simulink model "elevator"  (R2019b)
settings: Solver=FixedStepAuto  StartTime=0.0  StopTime=10.0  RelTol=1e-3
libraries: eePwmGenerator x2
settings Model: ExtModeTrigDuration=2  Creator=sin29  LastModifiedBy=mr
settings DataIOCC: ReturnWorkspaceOutputs=off
settings OptimizationCC: DefaultParameterBehavior=Inlined  UseDivisionForNetSlopeComputation=on  UseFloatMulNetSlope=on  InlineInvariantSignals=on  PassReuseOutputArgsAs=Individual arguments  ZeroExternalMemoryAtStartup=off  ZeroInternalMemoryAtStartup=off  NoFixptDivByZeroProtection=on  EfficientFloat2IntCast=on  LifeSpan=1  MaxStackSize=64  OptimizeBlockOrder=speed  DifferentSizesBufferReuse=on  EfficientTunableParamExpr=on
settings DebuggingCC: ParameterTunabilityLossMsg=error  ArithmeticOperatorsInVariantConditions=warning
settings HardwareCC: ProdBitPerInt=16  ProdBitPerPointer=16  ProdBitPerSizeT=16  ProdBitPerPtrDiffT=16  ProdLargestAtomicFloat=None  ProdWordSize=8  ProdLongLongMode=on  ProdHWDeviceType=Atmel->AVR
settings SFSimCC: MATLABDynamicMemAlloc=off  CustomCodeUndefinedFunction=UseInterfaceOnly
settings RTWCC: SystemTargetFile=ert.tlc  HardwareBoard=Arduino Uno  TLCOptions=-aInlineSetEventsForThisBaseRateFcn=TLC_FALSE -aSuppressMultiTaskScheduler=TLC_FALSE -aRateBasedStepFcn=1  GenCodeOnly=on  TemplateMakefile=ert_default_tmf  GenerateReport=on  Toolchain=Arduino AVR  BuildConfiguration=Faster Runs  IncludeHyperlinkInReport=on  LaunchReport=on  GenerateTraceInfo=on  GenerateTraceReport=on  GenerateTraceReportSl=on  GenerateTraceReportSf=on  GenerateTraceReportEml=on  GenerateCodeMetricsReport=on
settings CodeAppCC: ForceParamTrailComments=on  IgnoreCustomStorageClasses=off  OperatorAnnotations=on  SimulinkDataObjDesc=on  SFDataObjDesc=on  CustomSymbolStrGlobalVar=rt$N$M  CustomSymbolStrType=$N$M  CustomSymbolStrFcn=$N$M$F  CustomSymbolStrMacro=$N$M  InsertBlockDesc=on
settings ERTTargetCC: IncludeMdlTerminateFcn=off  CombineSignalStateStructs=on  SupportAbsoluteTime=off  SupportComplex=off  SupportNonInlinedSFcns=on  InlinedParameterPlacement=NonHierarchical  ERTFilePackagingFormat=CompactWithDataFile

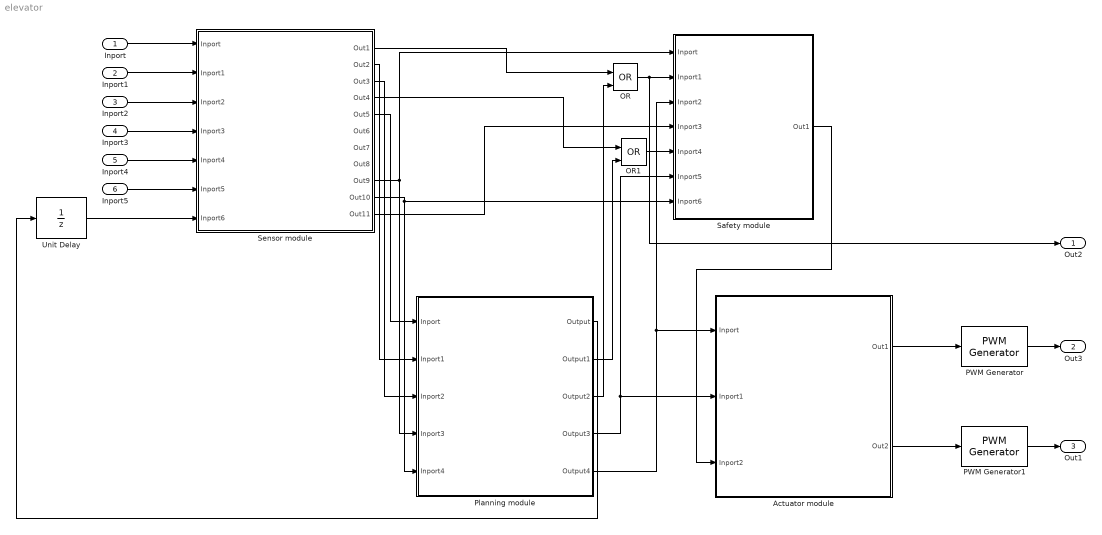
== system elevator ==
  Inport : Inport
  Inport1 : Inport  Port=2
  Inport2 : Inport  Port=3
  Inport3 : Inport  Port=4
  Inport4 : Inport  Port=5
  Inport5 : Inport  Port=6
  Actuator module : Subsystem
  OR : Logic  Operator=OR  IconShape=distinctive  AllPortsSameDT=off  OutDataTypeStr=boolean
  OR1 : Logic  Operator=OR  IconShape=distinctive  AllPortsSameDT=off  OutDataTypeStr=boolean
  PWM Generator : eePwmGenerator/PWM Generator  CarrCount=Up  Tper=0.001  Ts=5e-5
      settings: SourceProductName=Simscape Electrical
  PWM Generator1 : eePwmGenerator/PWM Generator  CarrCount=Up  Tper=0.001  Ts=5e-5
      settings: SourceProductName=Simscape Electrical
  Planning module : Subsystem
  Safety module : Subsystem
  Sensor module : Subsystem
  Unit Delay : UnitDelay  SampleTime=-1  HasFrameUpgradeWarning=on
  Out2 : Outport
  Out3 : Outport  Port=2
  Out1 : Outport  Port=3
  wires:
  Inport3/1 -> Sensor module/4(Inport3)
  Inport4/1 -> Sensor module/5(Inport4)
  Inport5/1 -> Sensor module/6(Inport5)
  Inport1/1 -> Sensor module/2(Inport1)
  Inport/1 -> Sensor module/1(Inport)
  Inport2/1 -> Sensor module/3(Inport2)
  Sensor module/4(Out4) -> OR1/1
  Sensor module/5(Out5) -> Planning module/1(Inport)
  Sensor module/2(Out2) -> Planning module/2(Inport1)
  Sensor module/3(Out3) -> Planning module/3(Inport2)
  Sensor module/10(Out10) -> Safety module/7(Inport6), Planning module/5(Inport4)
  Sensor module/9(Out9) -> Safety module/1(Inport), Planning module/4(Inport3)
  Unit Delay/1 -> Sensor module/7(Inport6)
  Planning module/1(Output) -> Unit Delay/1
  Sensor module/11(Out11) -> Safety module/4(Inport3)
  Sensor module/1(Out1) -> OR/1
  OR/1 -> Safety module/2(Inport1), Out2/1
  Planning module/3(Output2) -> OR/2
  OR1/1 -> Safety module/5(Inport4)
  Planning module/2(Output1) -> OR1/2
  Planning module/4(Output3) -> Actuator module/2(Inport1), Safety module/6(Inport5)
  Planning module/5(Output4) -> Actuator module/1(Inport), Safety module/3(Inport2)
  PWM Generator/1 -> Out3/1
  PWM Generator1/1 -> Out1/1
  Safety module/1(Out1) -> Actuator module/3(Inport2)
  Actuator module/1(Out1) -> PWM Generator/1
  Actuator module/2(Out2) -> PWM Generator1/1

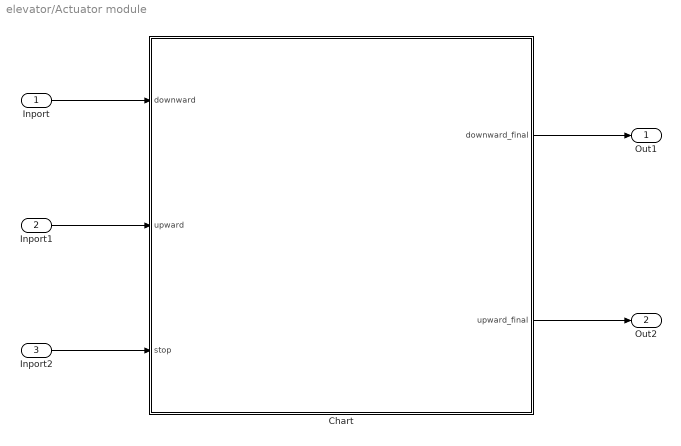
== system elevator/Actuator module ==
  Inport : Inport
  Inport1 : Inport  Port=2
  Inport2 : Inport  Port=3
  Chart : Stateflow chart  BlockKeywords=__PRM__SERIALIZED__DATA__:Stateflow Chart,Stateflow Diagram  TreatAsAtomicUnit=on
  Out1 : Outport
  Out2 : Outport  Port=2
  wires:
  Inport/1 -> Chart/1(downward)
  Inport1/1 -> Chart/2(upward)
  Inport2/1 -> Chart/3(stop)
  Chart/1(downward_final) -> Out1/1
  Chart/2(upward_final) -> Out2/1

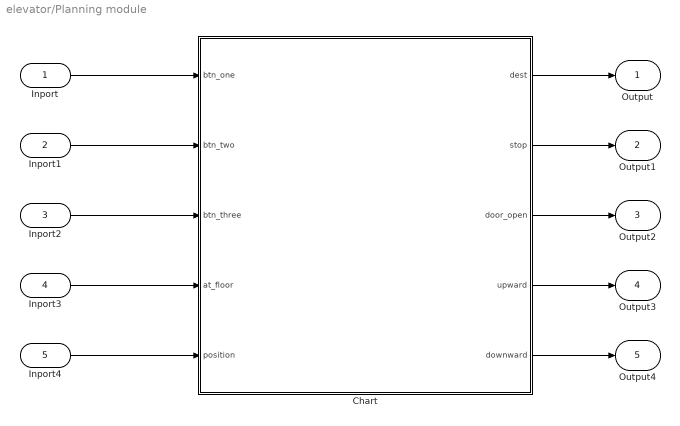
== system elevator/Planning module ==
  Inport : Inport
  Inport1 : Inport  Port=2
  Inport2 : Inport  Port=3
  Inport3 : Inport  Port=4
  Inport4 : Inport  Port=5
  Chart : Stateflow chart  BlockKeywords=__PRM__SERIALIZED__DATA__:Stateflow Chart,Stateflow Diagram  TreatAsAtomicUnit=on
  Output : Outport
  Output1 : Outport  Port=2
  Output2 : Outport  Port=3
  Output3 : Outport  Port=4
  Output4 : Outport  Port=5
  wires:
  Inport/1 -> Chart/1(btn_one)
  Inport4/1 -> Chart/5(position)
  Inport3/1 -> Chart/4(at_floor)
  Inport2/1 -> Chart/3(btn_three)
  Inport1/1 -> Chart/2(btn_two)
  Chart/1(dest) -> Output/1
  Chart/2(stop) -> Output1/1
  Chart/3(door_open) -> Output2/1
  Chart/5(downward) -> Output4/1
  Chart/4(upward) -> Output3/1

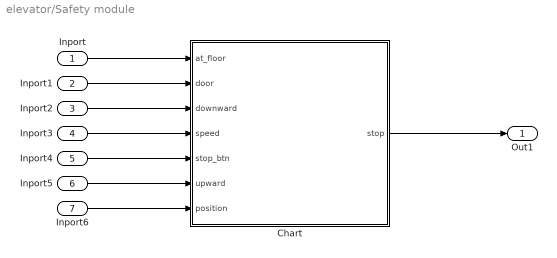
== system elevator/Safety module ==
  Inport : Inport
  Inport1 : Inport  Port=2
  Inport2 : Inport  Port=3
  Inport3 : Inport  Port=4
  Inport4 : Inport  Port=5
  Inport5 : Inport  Port=6
  Inport6 : Inport  Port=7
  Chart : Stateflow chart  TreatAsAtomicUnit=on
  Out1 : Outport  VectorParamsAs1DForOutWhenUnconnected=off
  wires:
  Inport/1 -> Chart/1(at_floor)
  Inport1/1 -> Chart/2(door)
  Inport2/1 -> Chart/3(downward)
  Inport3/1 -> Chart/4(speed)
  Inport4/1 -> Chart/5(stop_btn)
  Inport5/1 -> Chart/6(upward)
  Chart/1(stop) -> Out1/1
  Inport6/1 -> Chart/7(position)

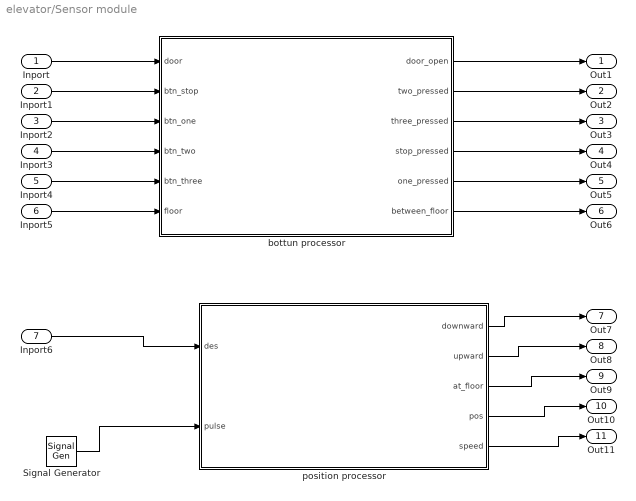
== system elevator/Sensor module ==
  Inport : Inport
  Inport1 : Inport  Port=2
  Inport2 : Inport  Port=3
  Inport3 : Inport  Port=4
  Inport4 : Inport  Port=5
  Inport5 : Inport  Port=6
  Inport6 : Inport  Port=7
  Signal Generator : SignalGenerator  Units=rad/sec
  "bottun processor " : Stateflow chart  TreatAsAtomicUnit=on
  "position processor " : Stateflow chart  TreatAsAtomicUnit=on
  Out1 : Outport  VectorParamsAs1DForOutWhenUnconnected=off
  Out2 : Outport  Port=2  VectorParamsAs1DForOutWhenUnconnected=off
  Out3 : Outport  Port=3  VectorParamsAs1DForOutWhenUnconnected=off
  Out4 : Outport  Port=4  VectorParamsAs1DForOutWhenUnconnected=off
  Out5 : Outport  Port=5  VectorParamsAs1DForOutWhenUnconnected=off
  Out6 : Outport  Port=6  VectorParamsAs1DForOutWhenUnconnected=off
  Out7 : Outport  Port=7  VectorParamsAs1DForOutWhenUnconnected=off
  Out8 : Outport  Port=8  VectorParamsAs1DForOutWhenUnconnected=off
  Out9 : Outport  Port=9  VectorParamsAs1DForOutWhenUnconnected=off
  Out10 : Outport  Port=10  VectorParamsAs1DForOutWhenUnconnected=off
  Out11 : Outport  Port=11  VectorParamsAs1DForOutWhenUnconnected=off
  wires:
  Inport/1 -> "bottun processor "/1(door)
  Inport1/1 -> "bottun processor "/2(btn_stop)
  Inport2/1 -> "bottun processor "/3(btn_one)
  Inport3/1 -> "bottun processor "/4(btn_two)
  Inport4/1 -> "bottun processor "/5(btn_three)
  Inport5/1 -> "bottun processor "/6(floor)
  Inport6/1 -> "position processor "/1(des)
  Signal Generator/1 -> "position processor "/2(pulse)
  "bottun processor "/1(door_open) -> Out1/1
  "bottun processor "/2(two_pressed) -> Out2/1
  "bottun processor "/3(three_pressed) -> Out3/1
  "bottun processor "/4(stop_pressed) -> Out4/1
  "bottun processor "/5(one_pressed) -> Out5/1
  "bottun processor "/6(between_floor) -> Out6/1
  "position processor "/1(downward) -> Out7/1
  "position processor "/2(upward) -> Out8/1
  "position processor "/3(at_floor) -> Out9/1
  "position processor "/4(pos) -> Out10/1
  "position processor "/5(speed) -> Out11/1

== stateflow chart elevator/Sensor module/position processor  ==
  state pos_detection
    state speed_cal [parallel]
      settings: executionOrder=1
      state speed_at_1
        entry:
        speed = (pos  - last_counter);
        last_counter = pos;
      (default) -> speed_at_1
      speed_at_1 -> speed_at_1 : [after(1,sec)]
    state pos_cal [parallel]
      settings: executionOrder=2
      (history)
      state floor_1
        entry:
        counter = 0;
        at_floor = 1;
        pos = 0;
        during:
        upward = 0;
        downward = 0;
      state floor_3
        entry:
        counter = 0;
        at_floor = 3;
        pos = 800;
        during:
        upward = 0;
        downward = 0;
      state between_1_2
        entry:
        at_floor = -1;
        pos = (upward)*(counter) + (downward)*(400 - counter)
        exit:
      state between_2_3
        entry:
        at_floor = -1;
        pos = (upward)*(counter+400) + (downward)*(800 - counter)
      state read_pulse_2_3
        entry:
        counter = counter+1
        last = pulse;
      state read_pulse_1_2
        entry:
        counter = counter+1
        last = pulse
      state floor_2
        entry:
        counter = 0;
        at_floor = 2;
        pos  = 400;
        during:
        upward = 0;
        downward = 0;
      read_pulse_1_2 -> floor_1 [order 1] : [counter == 400 && downward == 1]
      read_pulse_2_3 -> floor_3 [order 1] : [counter == 400 && upward == 1]
      floor_1 -> between_1_2 : [des == 2 || des == 3]{upward = 1;downward = 0}
      floor_3 -> between_2_3 : [des == 2 || des == 1]{upward = 0 ; downward = 1}
      between_1_2 -> between_1_2 [order 2] : [after(3,msec)&&last == pulse]
      read_pulse_1_2 -> between_1_2 [order 3] : [counter ~= 400]
      floor_2 -> between_2_3 [order 2] : [des == 3]{upward = 1; downward = 0}
      read_pulse_2_3 -> between_2_3 [order 3] : [counter ~= 400]
      between_2_3 -> read_pulse_2_3 : [after(3,msec)&& last ~= pulse]
      between_1_2 -> read_pulse_1_2 [order 1] : [after(3,msec)&& last ~= pulse]
      floor_2 -> between_1_2 [order 1] : [des == 1]{upward = 0;downward =1;}
      read_pulse_2_3 -> floor_2 [order 2] : [counter == 400 && downward == 1]
      read_pulse_1_2 -> floor_2 [order 2] : [counter == 400 && upward == 1]
    (default) -> floor_1
  state init
    exit :
    counter = 0;
    last_counter = 0;
    pos = 0;
  (default) -> init
  init -> pos_detection
  data: des input; pulse input; counter local; downward output; upward output; last local; at_floor output; pos output; speed output; last_counter local

== stateflow chart elevator/Safety module/Chart ==
  state down_stop
    entry :
    stop = 1;
  state both_dir_stop
    entry:
    stop = 1;
  state monitor
    during:
    stop = 0;
  state door_stop
    entry :
    stop = 1;
  state stop_button
    entry :
    stop = 1;
  state speed_stop
    entry :
    stop = 1;
  state top_stop
    entry :
    stop = 1;
  down_stop -> down_stop [order 1] : [after (10, msec) && position == 800 && at_floor == -1 && upward == 1]
  down_stop -> monitor [order 2] : [after (10, msec)  &&( at_floor ~= -1 || downward == 0)]
  monitor -> down_stop [order 5] : [after (10, msec) && position == 0 && at_floor == -1 && downward == 1]
  (default) -> monitor
  both_dir_stop -> both_dir_stop [order 2] : [after(10, msec) && upward == 1 && downward == 1]
  both_dir_stop -> monitor [order 1] : [after(10, msec) && (upward == 0 || downward == 0)]
  monitor -> both_dir_stop [order 6] : [after(10, msec) && upward == 1 && downward == 1]
  monitor -> top_stop [order 3] : [after (10, msec) && position == 800 && at_floor == -1 && upward == 1]
  monitor -> door_stop [order 1] : [after(10, msec) && door == 1 && at_floor ==-1]
  door_stop -> monitor [order 2] : [after(3, msec) && door == 0]
  top_stop -> monitor [order 1] : [after (10, msec)  &&( at_floor ~= -1 || upward == 0)]
  monitor -> stop_button [order 2] : [after (10, msec) && stop_btn == 1]
  stop_button -> monitor [order 2] : [after(3, msec) && stop_btn == 0]
  speed_stop -> monitor [order 1] : [after (10, msec) && speed <= 50]
  monitor -> speed_stop [order 4] : [after (10, msec) && speed > 50]
  door_stop -> door_stop [order 1] : [after(3, msec) && door == 1]
  stop_button -> stop_button [order 1] : [after(3, msec) && stop_btn == 1]
  speed_stop -> speed_stop [order 2] : [after (10, msec) && speed > 50]
  top_stop -> top_stop [order 2] : [after (10, msec) && position == 800 && at_floor == -1 && upward == 1]
  data: at_floor input; door input; downward input; speed input; stop_btn input; upward input; stop output; position input

== stateflow chart elevator/Sensor module/bottun processor  ==
  state Reset
    entry:
    one_pressed = 0;
    two_pressed = 0;
    three_pressed = 0;
    door_open = 0;
    stop_pressed = 0;
  state two_bounce
  state three_bounce
  state stop_bounce
  state one_bounce
  state door_bounce
  state floor_bounce
  state floor_pos
    entry :
    between_floor = 1;
  state two_press
    entry:
    two_pressed = 1;
  state stop_press
    entry:
    stop_pressed =1 ;
  state three_press
    entry:
    three_pressed = 1;
  state door_status
    entry:
    door_open = 1;
  state one_press
    entry:
    one_pressed = 1;
  floor_pos -> Reset
  floor_bounce -> Reset [order 1] : [floor == 0]
  Reset -> floor_bounce [order 6] : [floor == 1]
  (default) -> Reset
  stop_press -> Reset
  one_press -> Reset
  Reset -> one_bounce [order 5] : [btn_one == 1]
  stop_bounce -> Reset [order 2] : [btn_stop == 0]
  one_bounce -> Reset [order 2] : [btn_one == 0]
  two_bounce -> Reset [order 2] : [btn_two == 0]
  Reset -> stop_bounce [order 4] : [btn_stop == 1]
  Reset -> two_bounce [order 1] : [btn_two == 1]
  door_bounce -> Reset [order 2] : [door == 0]
  two_press -> Reset
  three_bounce -> Reset [order 2] : [btn_three == 0]
  Reset -> three_bounce [order 2] : [btn_three== 1]
  three_press -> Reset
  door_status -> Reset
  Reset -> door_bounce [order 3] : [door == 1]
  two_bounce -> two_press [order 1] : [btn_two == 1&&after(0.2,msec)]
  three_bounce -> three_press [order 1] : [btn_three == 1&&after(0.2,msec)]
  stop_bounce -> stop_press [order 1] : [btn_stop == 1&&after(0.2,msec)]
  one_bounce -> one_press [order 1] : [btn_one == 1&&after(0.2,msec)]
  door_bounce -> door_status [order 1] : [door == 1&&after(0.2,msec)]
  floor_bounce -> floor_pos [order 2] : [floor == 1&&after(0.2,msec)]
  data: door input; btn_stop input; door_open output; two_pressed output; three_pressed output; stop_pressed output; one_pressed output; btn_one input; btn_two input; btn_three input; between_floor output; floor input

== stateflow chart elevator/Planning module/Chart ==
  state planning_cal
    state plan_handle [parallel]
      settings: executionOrder=1
      state floor1
        entry:
        one_pressed = 0;
        door_open = 1;
        stop = 1;
      state floor3
        entry:
        three_pressed = 0;
        door_open = 1;
        stop = 1;
      state move_up
        entry:
        door_open = 0;
        stop = 0;
        upward = 1;
        downward = 0;
      state move_down
        entry:
        door_open = 0;
        stop = 0;
        upward = 0;
        downward = 1;
      state floor2
        entry:
        two_pressed = 0;
        door_open = 1;
        stop = 1;
      floor1 -> floor1 [order 1] : [one_pressed == 1]
      (default) -> floor1
      floor1 -> move_up [order 2] : [after(5, sec) && two_pressed == 1]{dest = 2; two_open = 1}
      move_down -> floor1 [order 3] : [one_pressed == 1 && at_floor == 1]
      floor1 -> move_up [order 3] : [after(5, sec) && two_pressed == 0 && three_pressed == 1]{dest = 3; two_open = 0}
      floor3 -> floor3 [order 1] : [three_pressed == 1]
      move_up -> move_up [order 1] : [two_pressed == 1 && two_open == 0 && position <= 200]{two_open = 1; dest = 2}
      move_up -> floor3 [order 3] : [three_pressed == 1 && at_floor == 3]
      floor3 -> move_down [order 2] : [after(5, sec) && two_pressed == 0 && one_pressed == 1]{dest = 1; two_open = 0}
      floor3 -> move_down [order 3] : [after(5, sec) && two_pressed == 1]{dest = 2; two_open = 1}
      floor2 -> move_up [order 2] : [after(5, sec) && three_pressed == 1]{dest = 3}
      move_up -> floor2 [order 2] : [at_floor == 2 && two_pressed == 1 && two_open == 1]
      floor2 -> floor2 [order 1] : [two_pressed == 1]
      move_down -> floor2 [order 1] : [at_floor == 2 && two_pressed == 1 && two_open == 1]
      move_down -> move_down [order 2] : [two_pressed == 1 && two_open == 0 && position >= 600]{two_open = 1; dest = 2}
      floor2 -> move_down [order 3] : [after(5, sec) && one_pressed == 1]{dest = 1}
    state btn_handle [parallel]
      settings: executionOrder=2
      state btn_handle
      (default) -> planning_cal.btn_handle.btn_handle
      planning_cal.btn_handle.btn_handle -> planning_cal.btn_handle.btn_handle [order 1] : [btn_two == 1]{two_pressed = 1}
      planning_cal.btn_handle.btn_handle -> planning_cal.btn_handle.btn_handle [order 3] : [btn_one == 1]{one_pressed = 1}
      planning_cal.btn_handle.btn_handle -> planning_cal.btn_handle.btn_handle [order 2] : [btn_three == 1]{three_pressed = 1}
  state init
    exit:
    one_pressed = 0;
    two_pressed = 0;
    three_pressed = 0;
  (default) -> init
  init -> planning_cal
  data: dest output; btn_one input; btn_two input; btn_three input; stop output; two_open local; door_open output; at_floor input; position input; one_pressed local; two_pressed local; three_pressed local; upward output; downward output

== stateflow chart elevator/Actuator module/Chart ==
  state stop
    entry:
    upward_final = 0;
    downward_final = 0;
  state move
    entry:
    upward_final = upward*0.5;
    downward_final = downward*0.5;
  (default) -> move
  move -> stop : [stop == 1]
  stop -> move : [stop == 0]
  data: downward input; upward input; downward_final output; upward_final output; stop input
